simulink model "SOHO_sim_UKF"  (R2018b)
settings: Solver=ode4  StartTime=0.0  StopTime=end_time  FixedStep=dt  RelTol=1e-8  AbsTol=1e-10
undefined symbols (not defined in the file or in its folder): A_RW, acc_gyro, areas, Astar_RW, att_det_method, bcs, DCM, dt, dt_UKF, gyro_noise, I_vec, I_w, mu, mu1, normals, omega, r0, Rot, RW_noise, star_err_var, star_noise, sun_err_var, sun_noise, v0, w0
libraries: sharedutil x1
settings Model: Creator=ayotundedemuren  LastModifiedBy=Ethan
settings SolverCC: AutoScaleAbsTol=off
settings DebuggingCC: UnderSpecifiedDimensionMsg=error

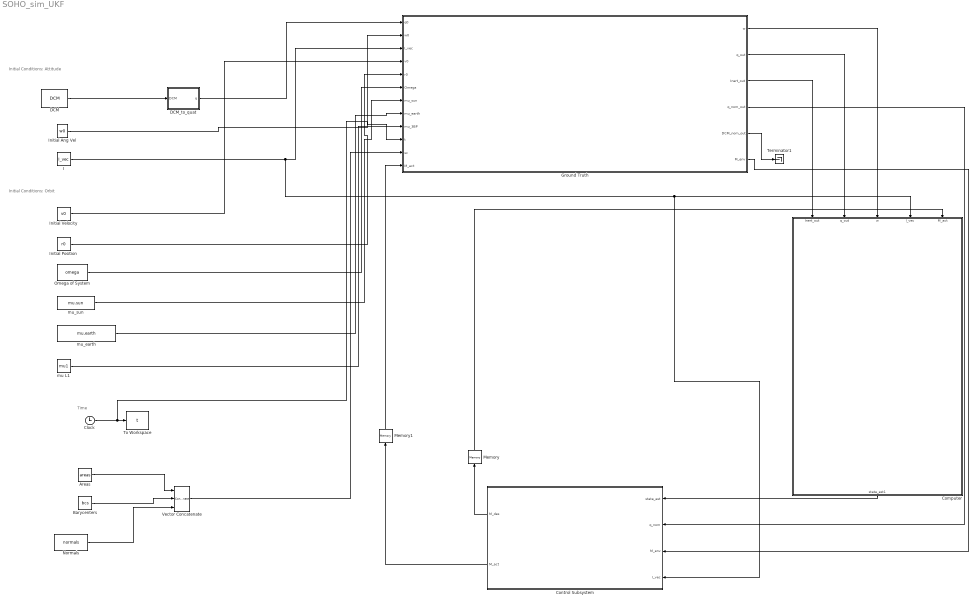
== system SOHO_sim_UKF ==
  note: Time
  note: Initial Conditions: Orbit
  note: Initial Conditions: Attitude
  Areas : Constant  Value=areas
  Barycenters : Constant  Value=bcs
  Clock : Clock
      settings: Decimation=100
  Computer : Subsystem
  Control Subsystem : Subsystem
  DCM : Constant  Value=DCM
  DCM_to_quat : MATLAB Function  TreatAsAtomicUnit=on
  Ground Truth : Subsystem
  I : Constant  Value=I_vec
  Initial Ang Vel : Constant  Value=w0
  Initial Position : Constant  Value=r0
  Initial Velocity : Constant  Value=v0
  Memory : Memory  InitialCondition=zeros(3,1)
  Memory1 : Memory  InitialCondition=zeros(3,1)
  Normals : Constant  Value=normals
  Omega of System : Constant  Value=omega
  Terminator1 : Terminator
  To Workspace : ToWorkspace  VariableName=t  SampleTime=-1
      settings: Save2DSignal=2-D array (concatenate along first dimension)
  Vector Concatenate : Concatenate  NumInputs=3  Mode=Multidimensional array  ConcatenateDimension=2
  mu L1 : Constant  Value=mu1
  mu_earth : Constant  Value=mu.earth
  mu_sun : Constant  Value=mu.sun
  wires:
  Normals/1 -> Vector Concatenate/3
  Barycenters/1 -> Vector Concatenate/2
  Areas/1 -> Vector Concatenate/1
  Clock/1 -> Ground Truth/10(t), To Workspace/1
  DCM/1 -> DCM_to_quat/1(DCM)
  DCM_to_quat/1(q) -> Ground Truth/1(q0)
  Initial Ang Vel/1 -> Ground Truth/2(w0)
  I/1 -> Control Subsystem/4(I_vec), Computer/4(I_vec), Ground Truth/3(I_vec)
  Initial Velocity/1 -> Ground Truth/4(v0)
  Initial Position/1 -> Ground Truth/5(r0)
  Omega of System/1 -> Ground Truth/6(Omega)
  mu_sun/1 -> Ground Truth/7(mu_sun)
  mu_earth/1 -> Ground Truth/8(mu_earth)
  mu L1/1 -> Ground Truth/9(mu_3BP)
  Vector Concatenate/1 -> Ground Truth/11(sc)
  Ground Truth/1(w) -> Computer/3(w)
  Ground Truth/2(q_out) -> Computer/2(q_out)
  Ground Truth/3(Inert_out) -> Computer/1(Inert_out)
  Ground Truth/5(DCM_nom_out) -> Terminator1/1
  Ground Truth/4(q_nom_out) -> Control Subsystem/2(q_nom)
  Control Subsystem/1(M_des) -> Memory/1
  Ground Truth/6(M_env) -> Control Subsystem/3(M_env)
  Memory/1 -> Computer/5(M_act)
  Control Subsystem/2(M_act) -> Memory1/1
  Memory1/1 -> Ground Truth/12(M_act)
  Computer/1(state_est1) -> Control Subsystem/1(state_est)

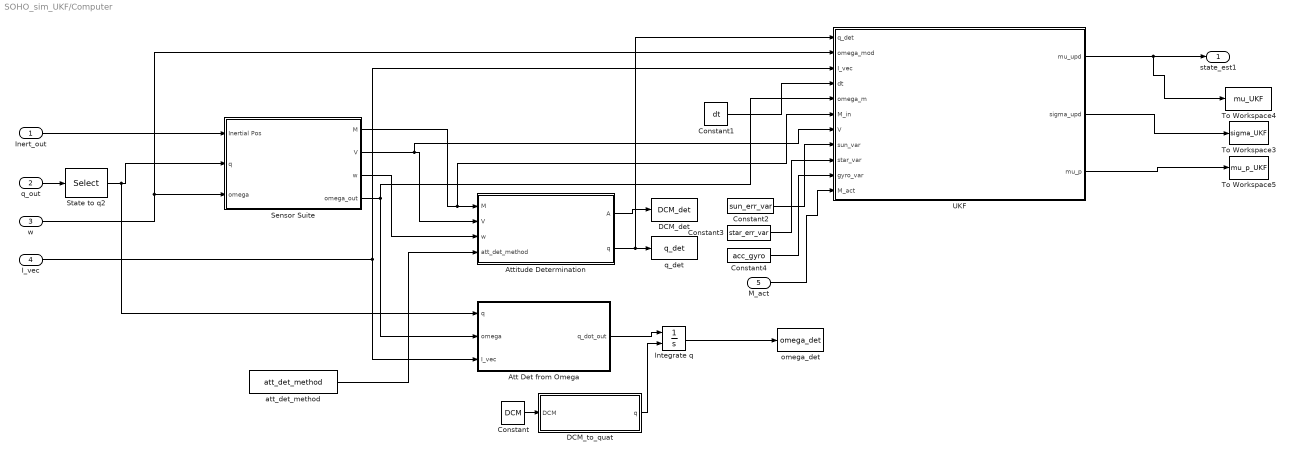
== system SOHO_sim_UKF/Computer ==
  Inert_out : Inport
  q_out : Inport  Port=2
  w : Inport  Port=3
  I_vec : Inport  Port=4
  M_act : Inport  Port=5
  Att Det from Omega : MATLAB Function  TreatAsAtomicUnit=on
  Attitude Determination : MATLAB Function  TreatAsAtomicUnit=on
  Constant : Constant  Value=DCM
  Constant1 : Constant  Value=dt
  Constant2 : Constant  Value=sun_err_var
  Constant3 : Constant  Value=star_err_var
  Constant4 : Constant  Value=acc_gyro
  DCM_det : ToWorkspace  VariableName=DCM_det  SampleTime=-1
  DCM_to_quat : MATLAB Function  TreatAsAtomicUnit=on
  Integrate q : Integrator  InitialConditionSource=external  InitialCondition=DCM(:)
  Sensor Suite : Subsystem
  State to q2 : Selector  InputPortWidth=7  IndexOptions=Starting index (dialog)  Indices=[1]  OutputSizes=4
  To Workspace3 : ToWorkspace  VariableName=sigma_UKF  SampleTime=-1
  To Workspace4 : ToWorkspace  VariableName=mu_UKF  SampleTime=-1
  To Workspace5 : ToWorkspace  VariableName=mu_p_UKF  SampleTime=-1
  UKF : MATLAB Function  TreatAsAtomicUnit=on  SystemSampleTime=dt_UKF
  att_det_method : Constant  Value=att_det_method
  omega_det : ToWorkspace  VariableName=omega_det  SampleTime=-1
  q_det : ToWorkspace  VariableName=q_det  SampleTime=-1
  state_est1 : Outport
  wires:
  Inert_out/1 -> Sensor Suite/1(Inertial Pos)
  q_out/1 -> State to q2/1
  Sensor Suite/1(M) -> UKF/6(M_in), Attitude Determination/1(M)
  Sensor Suite/2(V) -> UKF/7(V), Attitude Determination/2(V)
  att_det_method/1 -> Attitude Determination/4(att_det_method)
  Sensor Suite/3(w) -> Attitude Determination/3(w)
  w/1 -> UKF/2(omega_mod), Sensor Suite/3(omega)
  I_vec/1 -> UKF/3(I_vec), Att Det from Omega/3(I_vec)
  Sensor Suite/4(omega_out) -> UKF/5(omega_m), Att Det from Omega/2(omega)
  Att Det from Omega/1(q_dot_out) -> Integrate q/1
  Attitude Determination/1(A) -> DCM_det/1
  Attitude Determination/2(q) -> UKF/1(q_det), q_det/1
  Constant/1 -> DCM_to_quat/1(DCM)
  DCM_to_quat/1(q) -> Integrate q/2
  Integrate q/1 -> omega_det/1
  State to q2/1 -> Att Det from Omega/1(q), Sensor Suite/2(q)
  Constant1/1 -> UKF/4(dt)
  Constant4/1 -> UKF/10(gyro_var)
  Constant3/1 -> UKF/9(star_var)
  Constant2/1 -> UKF/8(sun_var)
  M_act/1 -> UKF/11(M_act)
  UKF/2(sigma_upd) -> To Workspace3/1
  UKF/3(mu_p) -> To Workspace5/1
  UKF/1(mu_upd) -> To Workspace4/1, state_est1/1

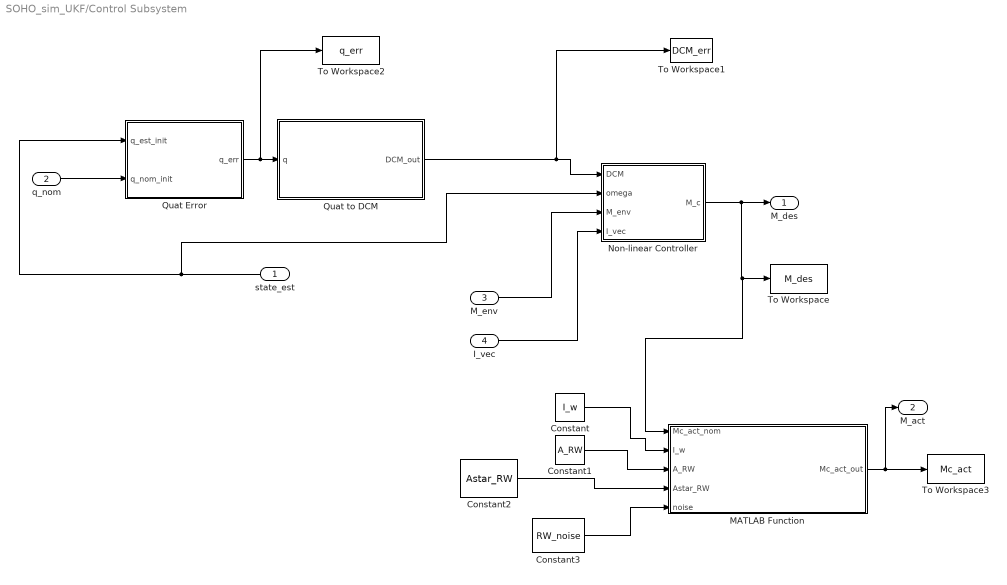
== system SOHO_sim_UKF/Control Subsystem ==
  state_est : Inport
  q_nom : Inport  Port=2
  M_env : Inport  Port=3
  I_vec : Inport  Port=4
  Constant : Constant  Value=I_w
  Constant1 : Constant  Value=A_RW
  Constant2 : Constant  Value=Astar_RW
  Constant3 : Constant  Value=RW_noise
  MATLAB Function : MATLAB Function  TreatAsAtomicUnit=on
  Non-linear Controller : MATLAB Function  TreatAsAtomicUnit=on
  Quat Error : MATLAB Function  TreatAsAtomicUnit=on
  Quat to DCM : MATLAB Function  TreatAsAtomicUnit=on
  To Workspace : ToWorkspace  VariableName=M_des  SampleTime=-1
  To Workspace1 : ToWorkspace  VariableName=DCM_err  SampleTime=-1
  To Workspace2 : ToWorkspace  VariableName=q_err  SampleTime=-1
  To Workspace3 : ToWorkspace  VariableName=Mc_act  SampleTime=-1
  M_des : Outport
  M_act : Outport  Port=2
  wires:
  q_nom/1 -> Quat Error/2(q_nom_init)
  state_est/1 -> Non-linear Controller/2(omega), Quat Error/1(q_est_init)
  Quat Error/1(q_err) -> To Workspace2/1, Quat to DCM/1(q)
  Non-linear Controller/1(M_c) -> MATLAB Function/1(Mc_act_nom), To Workspace/1, M_des/1
  Quat to DCM/1(DCM_out) -> To Workspace1/1, Non-linear Controller/1(DCM)
  M_env/1 -> Non-linear Controller/3(M_env)
  I_vec/1 -> Non-linear Controller/4(I_vec)
  MATLAB Function/1(Mc_act_out) -> M_act/1, To Workspace3/1
  Constant/1 -> MATLAB Function/2(I_w)
  Constant1/1 -> MATLAB Function/3(A_RW)
  Constant2/1 -> MATLAB Function/4(Astar_RW)
  Constant3/1 -> MATLAB Function/5(noise)

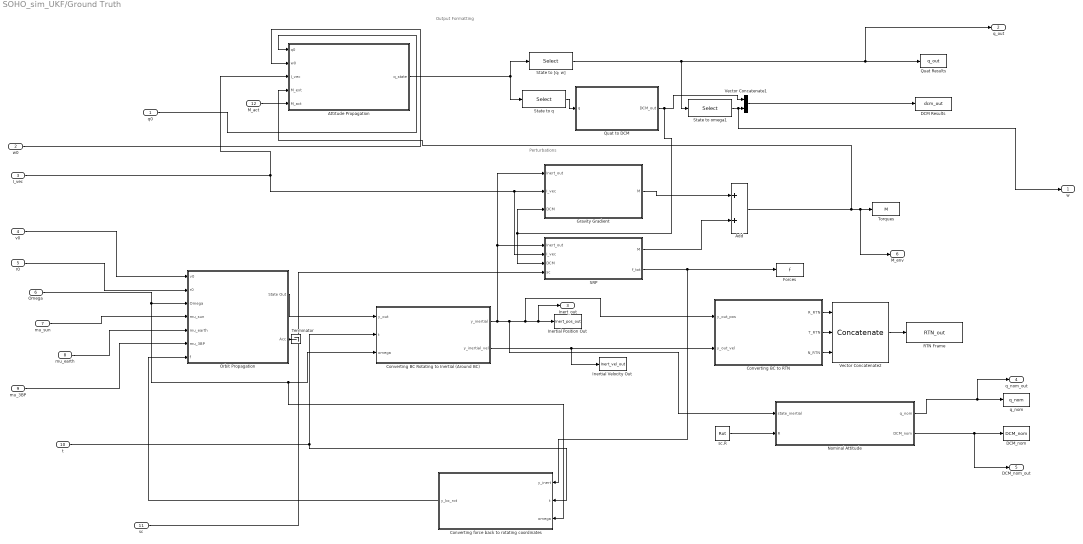
== system SOHO_sim_UKF/Ground Truth ==
  note: Perturbations
  note: Output Formatting
  q0 : Inport
  w0 : Inport  Port=2
  I_vec : Inport  Port=3
  v0 : Inport  Port=4
  r0 : Inport  Port=5
  Omega : Inport  Port=6
  mu_sun : Inport  Port=7
  mu_earth : Inport  Port=8
  mu_3BP : Inport  Port=9
  t : Inport  Port=10
  sc : Inport  Port=11
  M_act : Inport  Port=12
  Add : Sum
  Attitude Propagation : Subsystem
  Converting BC Rotating to Inertial (Around BC) : MATLAB Function  TreatAsAtomicUnit=on
  Converting BC to RTN : MATLAB Function  TreatAsAtomicUnit=on
  Converting force back to rotating coordinates : MATLAB Function  TreatAsAtomicUnit=on
  DCM Results : ToWorkspace  VariableName=dcm_out  SampleTime=-1
      settings: Save2DSignal=2-D array (concatenate along first dimension)
  DCM_nom : ToWorkspace  VariableName=DCM_nom  SampleTime=-1
  Forces : ToWorkspace  VariableName=f  SampleTime=-1
  Gravity Gradient : MATLAB Function  TreatAsAtomicUnit=on
  Inertial Position Out : ToWorkspace  VariableName=Inert_pos_out  SampleTime=-1
  Inertial Velocity Out : ToWorkspace  VariableName=Inert_vel_out  SampleTime=-1
  Nominal Attitude : MATLAB Function  TreatAsAtomicUnit=on
  Orbit Propagation : Subsystem
  Quat Results : ToWorkspace  VariableName=q_out  SampleTime=-1
  Quat to DCM : MATLAB Function  TreatAsAtomicUnit=on
  RTN Frame : ToWorkspace  VariableName=RTN_out  SampleTime=-1
  SRP : MATLAB Function  TreatAsAtomicUnit=on
  State to [q; w] : Selector  InputPortWidth=10  IndexOptions=Starting index (dialog)  Indices=[1]  OutputSizes=7
  State to omega1 : Selector  InputPortWidth=7  IndexOptions=Starting index (dialog)  Indices=5  OutputSizes=3
  State to q : Selector  InputPortWidth=10  IndexOptions=Starting index (dialog)  Indices=[1]  OutputSizes=4
  Terminator : Terminator
  Torques : ToWorkspace  VariableName=M  SampleTime=-1
  Vector Concatenate1 : Concatenate
  Vector Concatenate2 : Concatenate  NumInputs=3  Mode=Multidimensional array  ConcatenateDimension=2
  q_nom : ToWorkspace  VariableName=q_nom  SampleTime=-1
  sc.R : Constant  Value=Rot
  w : Outport
  q_out : Outport  Port=2
  Inert_out : Outport  Port=3
  q_nom_out : Outport  Port=4
  DCM_nom_out : Outport  Port=5
  M_env : Outport  Port=6
  wires:
  Vector Concatenate2/1 -> RTN Frame/1
  State to [q; w]/1 -> State to omega1/1, q_out/1, Quat Results/1
  mu_sun/1 -> Orbit Propagation/4(mu_sun)
  Omega/1 -> Orbit Propagation/3(Omega), Converting force back to rotating coordinates/3(omega), Converting BC Rotating to Inertial (Around BC)/3(omega)
  Vector Concatenate1/1 -> DCM Results/1
  sc/1 -> SRP/4(sc)
  State to q/1 -> Quat to DCM/1(q)
  Quat to DCM/1(DCM_out) -> SRP/3(DCM), Gravity Gradient/3(DCM), Vector Concatenate1/1
  State to omega1/1 -> w/1, Vector Concatenate1/2
  r0/1 -> Orbit Propagation/2(r0)
  Nominal Attitude/1(q_nom) -> q_nom_out/1, q_nom/1
  I_vec/1 -> Attitude Propagation/3(I_vec), SRP/2(I_vec), Gravity Gradient/2(I_vec)
  Converting BC to RTN/1(R_RTN) -> Vector Concatenate2/1
  SRP/2(f_tot) -> Converting force back to rotating coordinates/1(y_inert), Forces/1
  Orbit Propagation/1(State Out) -> Converting BC Rotating to Inertial (Around BC)/1(y_out)
  t/1 -> Converting BC Rotating to Inertial (Around BC)/2(t), Converting force back to rotating coordinates/2(t)
  Converting BC Rotating to Inertial (Around BC)/1(y_inertial) -> SRP/1(Inert_out), Gravity Gradient/1(Inert_out), Nominal Attitude/1(state_inertial), Converting BC to RTN/1(y_out_pos), Inert_out/1, Inertial Position Out/1
  Converting BC Rotating to Inertial (Around BC)/2(y_inertial_vel) -> Inertial Velocity Out/1, Converting BC to RTN/2(y_out_vel)
  q0/1 -> Attitude Propagation/1(q0)
  Converting BC to RTN/2(T_RTN) -> Vector Concatenate2/2
  Converting force back to rotating coordinates/1(y_bc_rot) -> Orbit Propagation/7(f)
  sc.R/1 -> Nominal Attitude/2(R)
  Nominal Attitude/2(DCM_nom) -> DCM_nom_out/1, DCM_nom/1
  v0/1 -> Orbit Propagation/1(v0)
  SRP/1(M) -> Add/2
  Attitude Propagation/1(q_state) -> State to [q; w]/1, State to q/1
  Gravity Gradient/1(M) -> Add/1
  Converting BC to RTN/3(N_RTN) -> Vector Concatenate2/3
  w0/1 -> Attitude Propagation/2(w0)
  mu_3BP/1 -> Orbit Propagation/6(mu_3BP)
  mu_earth/1 -> Orbit Propagation/5(mu_earth)
  Orbit Propagation/2(Acc) -> Terminator/1
  Add/1 -> Attitude Propagation/4(M_ext), M_env/1, Torques/1
  M_act/1 -> Attitude Propagation/5(M_act)

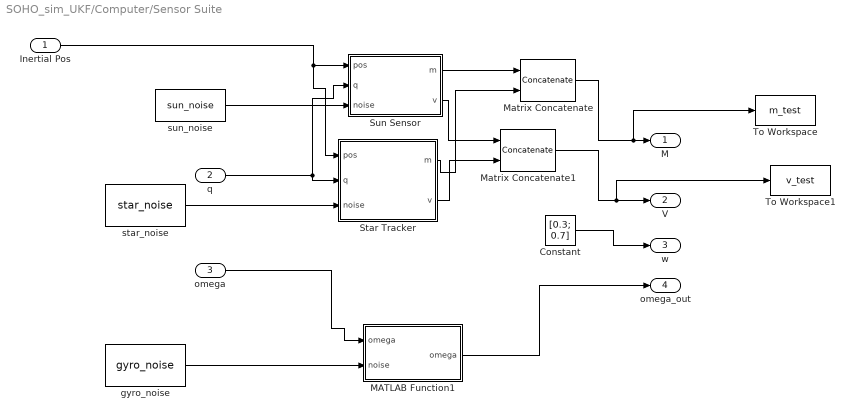
== system SOHO_sim_UKF/Computer/Sensor Suite ==
  Inertial Pos : Inport
  q : Inport  Port=2
  omega : Inport  Port=3
  Constant : Constant  Value=[0.3; 0.7]  VectorParams1D=off
  MATLAB Function1 : MATLAB Function  TreatAsAtomicUnit=on  SystemSampleTime=dt
  Matrix Concatenate : Concatenate  Mode=Multidimensional array  ConcatenateDimension=2
  Matrix Concatenate1 : Concatenate  Mode=Multidimensional array  ConcatenateDimension=2
  Star Tracker : MATLAB Function  TreatAsAtomicUnit=on  SystemSampleTime=dt
  Sun Sensor : MATLAB Function  TreatAsAtomicUnit=on  SystemSampleTime=dt
  To Workspace : ToWorkspace  VariableName=m_test  SampleTime=-1
  To Workspace1 : ToWorkspace  VariableName=v_test  SampleTime=-1
  gyro_noise : Constant  Value=gyro_noise  VectorParams1D=off
  star_noise : Constant  Value=star_noise  VectorParams1D=off
  sun_noise : Constant  Value=sun_noise  VectorParams1D=off
  M : Outport
  V : Outport  Port=2
  w : Outport  Port=3
  omega_out : Outport  Port=4
  wires:
  Inertial Pos/1 -> Star Tracker/1(pos), Sun Sensor/1(pos)
  q/1 -> Sun Sensor/2(q), Star Tracker/2(q)
  omega/1 -> MATLAB Function1/1("omega ")
  Sun Sensor/1(m) -> Matrix Concatenate/1
  Star Tracker/1(m) -> Matrix Concatenate/2
  Matrix Concatenate/1 -> To Workspace/1, M/1
  Sun Sensor/2(v) -> Matrix Concatenate1/1
  Star Tracker/2(v) -> Matrix Concatenate1/2
  Matrix Concatenate1/1 -> To Workspace1/1, V/1
  Constant/1 -> w/1
  MATLAB Function1/1(omega) -> omega_out/1
  sun_noise/1 -> Sun Sensor/3(noise)
  star_noise/1 -> Star Tracker/3(noise)
  gyro_noise/1 -> MATLAB Function1/2(noise)

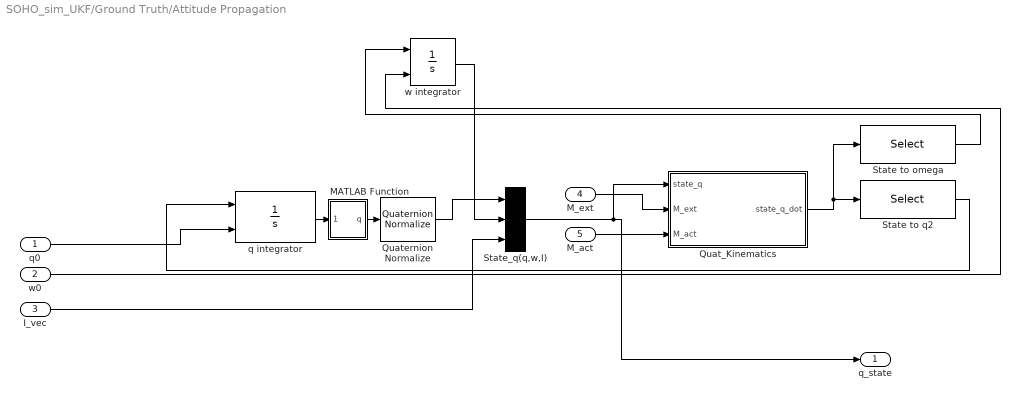
== system SOHO_sim_UKF/Ground Truth/Attitude Propagation ==
  q0 : Inport
  w0 : Inport  Port=2
  I_vec : Inport  Port=3
  M_ext : Inport  Port=4
  M_act : Inport  Port=5
  MATLAB Function : MATLAB Function  TreatAsAtomicUnit=on
  Quat_Kinematics : MATLAB Function  TreatAsAtomicUnit=on
  Quaternion Normalize : sharedutil/Quaternion Normalize  aMode=aMode
      settings: SourceProductName=Aerospace Blockset  SourceProductBaseCode=AE
  State to omega : Selector  InputPortWidth=10  IndexOptions=Starting index (dialog)  Indices=5  OutputSizes=3
  State to q2 : Selector  InputPortWidth=10  IndexOptions=Starting index (dialog)  Indices=[1]  OutputSizes=4
  State_q(q,w,I) : Concatenate  NumInputs=3
  q integrator : Integrator  InitialConditionSource=external
  w integrator : Integrator  InitialConditionSource=external
  q_state : Outport
  wires:
  State_q(q,w,I)/1 -> q_state/1, Quat_Kinematics/1(state_q)
  w integrator/1 -> State_q(q,w,I)/2
  State to omega/1 -> w integrator/1
  Quat_Kinematics/1(state_q_dot) -> State to omega/1, State to q2/1
  State to q2/1 -> q integrator/1
  w0/1 -> w integrator/2
  q0/1 -> q integrator/2
  I_vec/1 -> State_q(q,w,I)/3
  M_ext/1 -> Quat_Kinematics/2(M_ext)
  M_act/1 -> Quat_Kinematics/3(M_act)
  Quaternion Normalize/1 -> State_q(q,w,I)/1
  q integrator/1 -> MATLAB Function/1(q_in)
  MATLAB Function/1(q) -> Quaternion Normalize/1

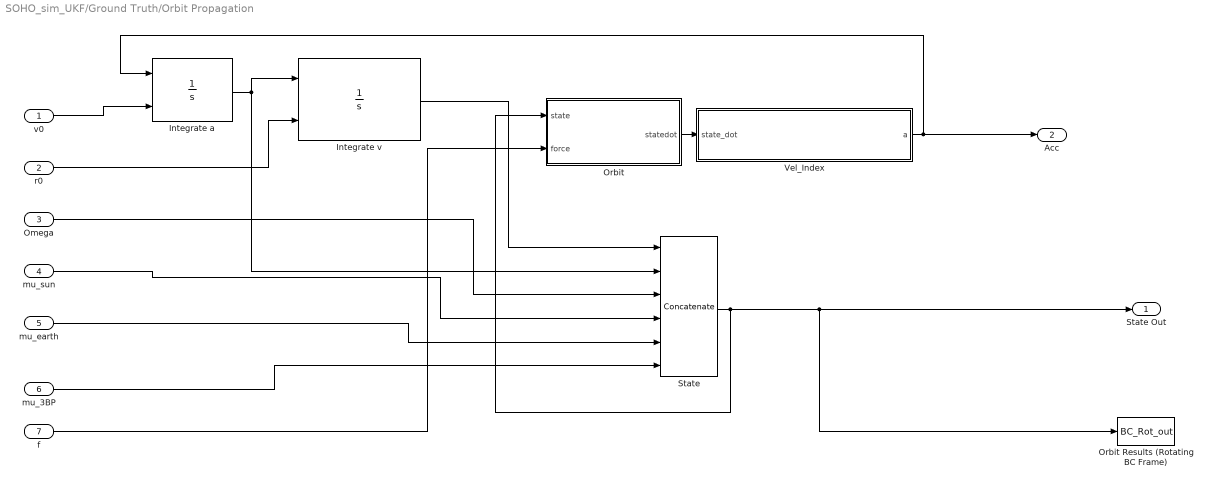
== system SOHO_sim_UKF/Ground Truth/Orbit Propagation ==
  v0 : Inport
  r0 : Inport  Port=2
  Omega : Inport  Port=3
  mu_sun : Inport  Port=4
  mu_earth : Inport  Port=5
  mu_3BP : Inport  Port=6
  f : Inport  Port=7
  Integrate a : Integrator  InitialConditionSource=external  AbsoluteTolerance=1e-6
  Integrate v : Integrator  InitialConditionSource=external  AbsoluteTolerance=1e-6
  Orbit : MATLAB Function  TreatAsAtomicUnit=on
  Orbit Results (Rotating BC Frame) : ToWorkspace  VariableName=BC_Rot_out  SampleTime=-1
  "State " : Concatenate  NumInputs=6
  Vel_Index : MATLAB Function  TreatAsAtomicUnit=on
  State Out : Outport
  Acc : Outport  Port=2
  wires:
  r0/1 -> Integrate v/2
  Integrate a/1 -> "State "/2, Integrate v/1
  Integrate v/1 -> "State "/1
  "State "/1 -> Orbit/1(state), Orbit Results (Rotating BC Frame)/1, State Out/1
  Vel_Index/1(a) -> Integrate a/1, Acc/1
  Orbit/1(statedot) -> Vel_Index/1(state_dot)
  v0/1 -> Integrate a/2
  mu_3BP/1 -> "State "/6
  Omega/1 -> "State "/3
  mu_sun/1 -> "State "/4
  mu_earth/1 -> "State "/5
  f/1 -> Orbit/2(force)

== matlab function SOHO_sim_UKF/Ground Truth/Orbit Propagation/Vel_Index ==
  data: state_dot input; a output
function a = fcn(state_dot)

a = state_dot(4:6);

end

== matlab function SOHO_sim_UKF/Ground Truth/Orbit Propagation/Orbit ==
  data: state input; statedot output; force input
function statedot = fcn(state, force)
force = force*0;
dis_sun = 149599650;

statedot = zeros(length(state),1);
x = state(1);
y = state(2);
z = state(3);
xdot = state(4);
ydot = state(5);
zdot = state(6);

w = state(7);
mu1 = state(8);
mu2 = state(9);
mu_sys = state(10);

Rx1 = - mu_sys*dis_sun;
Rx2 = (1-mu_sys)*dis_sun;

R1 = sqrt((x - Rx1)^2 + y^2 + z^2);
R2 = sqrt((x - Rx2)^2 + y^2 + z^2);

statedot(1) = xdot;
statedot(2) = ydot;
statedot(3) = zdot;

statedot(4) = x*w^2 + 2*ydot*w + mu1 * (Rx1 - x)/R1^3 + mu2 * (Rx2 - x)/R2^3 + force(1);
statedot(5) = y*w^2 - 2*xdot*w - mu1 * (y)/R1^3 - mu2 * (y)/R2^3 + force(2);
statedot(6) = - mu1 * (z)/R1^3 - mu2 * (z)/R2^3 + force(3);
end

== matlab function SOHO_sim_UKF/Ground Truth/Converting BC to RTN ==
  data: y_out_pos input; R_RTN output; T_RTN output; N_RTN output; y_out_vel input
function [R_RTN, T_RTN, N_RTN] = BCRot_to_RTN(y_out_pos, y_out_vel)
% 
% %% RTN Frame Rotating
% r = y_out(1:3);
% v = y_out(4:6);
% R_RTN = zeros(3,1);
% T_RTN = zeros(3,1);
% N_RTN = zeros(3,1);
% 
% for ii = 1:1
% 
%     R_RTN = r ./ norm(r);
%     N_RTN = cross(r,v) ./norm(cross(r,v));
%     T_RTN = cross(N_RTN, R_RTN) ./ norm(cross(N_RTN, R_RTN));
% end

%% RTN Frame Inertial
r = y_out_pos(1:3);
v = y_out_vel(1:3);
R_RTN = zeros(3,1);
T_RTN = zeros(3,1);
N_RTN = zeros(3,1);

for ii = 1:1

    R_RTN = r ./ norm(r);
    N_RTN = cross(r,v) ./norm(cross(r,v));
    T_RTN = cross(N_RTN, R_RTN) ./ norm(cross(N_RTN, R_RTN));
end
end

== matlab function SOHO_sim_UKF/Ground Truth/Converting BC Rotating to Inertial (Around BC) ==
  data: y_out input; y_inertial output; t input; omega input; y_inertial_vel output
function [y_inertial, y_inertial_vel] = BCRot_to_Inertial(y_out, t, omega)
wt = omega * t;
R = zeros(3,3);
R(1,:) = [cos(wt) sin(wt) 0];
R(2,:) = [-sin(wt) cos(wt) 0];
R(3,:) = [0 0 1];

sun_init = [-4.548476597303452e+02; 0; 0];
earth_init = [1.495991951523403e+08; 0; 0];
y_inertial = zeros(9, 1);
y_inertial_vel = zeros(9, 1);

y_inertial(1:3) = R' * y_out(1:3);
y_inertial_vel(1:3) = R' * y_out(4:6) + cross([0; 0; omega], y_inertial(1:3));
y_inertial(4:6) = R' * sun_init;
y_inertial_vel(4:6) = cross([0; 0; omega], y_inertial(4:6));
y_inertial(7:9) = R' * earth_init;
y_inertial_vel(7:9) = cross([0; 0; omega], y_inertial(7:9));
end

== matlab function SOHO_sim_UKF/Ground Truth/Attitude Propagation/Quat_Kinematics ==
  data: state_q input; state_q_dot output; M_ext input; M_act input
function state_q_dot  = quat_kin(state_q, M_ext, M_act)
% state = [q1 q2 q3 q4 w1 w2 w3 I1 I2 I3]

state_q_dot = zeros(length(state_q),1);
wx = state_q(5);
wy = state_q(6);
wz = state_q(7);
%% Kinematic Equations
Omega = [0 wz -wy wx; -wz 0 wx wy; wy -wx 0 wz; -wx -wy -wz 0];
err = 1 - norm(state_q(1:4));
state_q_dot(1:4) = 1/2 * Omega * state_q(1:4) + 0.05 * err * state_q(1:4);

%% Euler Equations
state_q_dot(5:end) = euler_eq(state_q(5:end), M_ext, M_act);
% state_q_dot(5) = -wy*wz * (state_q(10) - state_q(9))/state_q(8);
% state_q_dot(6) = -wx*wz * (state_q(8) - state_q(10))/state_q(9);
% state_q_dot(7) = -wx*wy * (state_q(9) - state_q(8))/state_q(10);

end

== matlab function SOHO_sim_UKF/DCM_to_quat ==
  data: DCM input; q output
function q  = DCM_to_quat(DCM)
B4 = 1/4 * (1 + trace(DCM));
B1 = 1/4 * (1 + 2*DCM(1,1) - trace(DCM));
B2 = 1/4 * (1 + 2*DCM(2,2) - trace(DCM));
B3 = 1/4 * (1 + 2*DCM(3,3) - trace(DCM));
B = [B1 B2 B3 B4];
[M, I] = max(B);
q = zeros(4,1);

q(I) = sqrt(B(I));
if I == 4
    q(1) = (DCM(2,3) - DCM(3,2)) / 4 / q(I);
    q(2) = (DCM(3,1) - DCM(1,3)) / 4 / q(I);
    q(3) = (DCM(1,2) - DCM(2,1)) / 4 / q(I);
elseif I == 3
  
    q(2) = (DCM(2,3) + DCM(3,2)) / 4 / q(I);
    q(1) = (DCM(3,1) + DCM(1,3)) / 4 / q(I);
    q(4) = (DCM(1,2) - DCM(2,1)) / 4 / q(I);
elseif I == 2

    q(3) = (DCM(2,3) + DCM(3,2)) / 4 / q(I);
    q(4) = (DCM(3,1) - DCM(1,3)) / 4 / q(I);
    q(1) = (DCM(1,2) + DCM(2,1)) / 4 / q(I);
elseif I == 1
    q(4) = (DCM(2,3) - DCM(3,2)) / 4 / q(I);
    q(3) = (DCM(3,1) + DCM(1,3)) / 4 / q(I);
    q(2) = (DCM(1,2) + DCM(2,1)) / 4 / q(I);
end
q = q/norm(q);
end

== matlab function SOHO_sim_UKF/Ground Truth/Gravity Gradient ==
  data: Inert_out input; M output; I_vec input; DCM input
function M = grav_grad(Inert_out, I_vec, DCM)
% Inert_out = [sat; sun; earth]

x = Inert_out(1);
y = Inert_out(2);
z = Inert_out(3);

x_s = Inert_out(4);
y_s = Inert_out(5);
z_s = Inert_out(6);

x_e = Inert_out(7);
y_e = Inert_out(8);
z_e = Inert_out(9);

Ix_sat = I_vec(1);
Iy_sat = I_vec(2);
Iz_sat = I_vec(3);

R_s = sqrt(((x - x_s).^2)+((y - y_s).^2)+((z - z_s).^2));
R_e = sqrt(((x - x_e).^2)+((y - y_e).^2)+((z - z_e).^2));

[A] = out2mat(DCM);
c_vec_s = A * [x-x_s; y-y_s; z-z_s];
cx_s = c_vec_s(1)/R_s;
cy_s = c_vec_s(2)/R_s;
cz_s = c_vec_s(3)/R_s;

c_vec_e = A * [x-x_e; y-y_e; z-z_e];
cx_e = c_vec_e(1)/R_e;
cy_e = c_vec_e(2)/R_e;
cz_e = c_vec_e(3)/R_e;

mu_earth = 3.986004418000000e+05;
mu_sun =  1.327124400180000e+11;

M_earth = (3*mu_earth./(R_e.^3)).*[((Iz_sat - Iy_sat).*cy_e.*cz_e)';...
    ((Ix_sat - Iz_sat).*cz_e.*cx_e)';...
    ((Iy_sat - Ix_sat).*cx_e.*cy_e)'];

M_sun = (3*mu_sun./(R_s.^3)).*[((Iz_sat - Iy_sat).*cy_s.*cz_s)';...
    ((Ix_sat - Iz_sat).*cz_s.*cx_s)';...
    ((Iy_sat - Ix_sat).*cx_s.*cy_s)'];

M = M_earth + M_sun;

== matlab function SOHO_sim_UKF/Ground Truth/Quat to DCM ==
  data: q input; DCM_out output
function DCM_out  = quat_to_DCM(q)

DCM = zeros(3, 3);
DCM(:, :) = ((q(4)^2 - norm(q(1:3))^2)*eye(3) ...
    + 2 * q(1:3) * q(1:3)'...
    - 2 * q(4) * ...
    [0, -q(3), q(2); q(3), 0, -q(1); ...
    -q(2), q(1), 0]);

DCM_out = DCM(:)';
end

== matlab function SOHO_sim_UKF/Ground Truth/Converting force back to rotating coordinates ==
  data: y_inert input; y_bc_rot output; t input; omega input
function y_bc_rot  = Inertial_to_BCRot(y_inert, t, omega)
wt = omega * t;
R = zeros(3,3);
R(1,:) = [cos(wt) sin(wt) 0];
R(2,:) = [-sin(wt) cos(wt) 0];
R(3,:) = [0 0 1];

y_bc_rot = zeros(3, 1);

y_bc_rot(1:3) = R * y_inert(1:3);

end

== matlab function SOHO_sim_UKF/Ground Truth/Nominal Attitude ==
  data: state_inertial input; q_nom output; DCM_nom output; R input
function [q_nom, DCM_nom] = nominal(state_inertial, R)
sat_pos = state_inertial(1:3);
sun_pos = state_inertial(4:6);

vect_to_sun = (sun_pos - sat_pos) / norm((sun_pos - sat_pos));
b_x = vect_to_sun;
b_y = cross([0; 0; 1], b_x);
b_z = cross(b_x, b_y);

DCM_nom_temp = R'*[b_x'; b_y'; b_z'];
q_nom = DCM_to_quat(DCM_nom_temp);

DCM_nom = DCM_nom_temp(:);


end

== matlab function SOHO_sim_UKF/Computer/Attitude Determination ==
  data: M input; A output; V input; w input; att_det_method input; q output
function [A, q] = att_det(M, V, w, att_det_method)

A = eye(3);
q = [0;0;0;1];
if att_det_method == 0
    A = det_method(M, V);
    q = DCM_to_quat(A);
    
elseif att_det_method == 1
    W = zeros(3, length(w));
    V2 = zeros(3, length(w));
    for ii = 1:length(w)
        W(:, ii) = sqrt(w(ii)).*M(:, ii);
        V2(:, ii) = sqrt(w(ii)).*V(:, ii);
    end
    [A, q] = q_method(W, V2);
    
elseif att_det_method == 2
    A = eye(3);
    q = ones(4,1);
end

end

== matlab function SOHO_sim_UKF/Computer/Sensor Suite/Sun Sensor ==
  data: pos input; m output; q input; v output; noise input
function [m, v] = sun_sens(pos, q, noise)
% Basic sun sensor
persistent count;
if isempty(count)
    count = 1;
elseif count >= size(noise, 2)
    count = 1;
    noise = [noise(3,:); -noise(1, :); noise(2, :)];
end


q = q(1:4);
A = quat_to_DCM(q);
v = (pos(4:6) - pos(1:3)) / norm((pos(4:6) - pos(1:3))); % sun to sat vec
m = A * v + noise(:, count); % currently this will give the exact measurement back 
count = count + 1;

end

== matlab function SOHO_sim_UKF/Computer/Att Det from Omega ==
  data: q input; omega input; q_dot_out output; I_vec input
function q_dot_out = fcn(q, omega, I_vec)
A = quat_to_DCM(q);
state = [q; omega; I_vec];
t = 1;
[state_dot] = quat_kin(t, state);
q_dot_out = state_dot(1:4);
end

== matlab function SOHO_sim_UKF/Computer/Sensor Suite/Star Tracker ==
  data: pos input; m output; q input; v output; noise input
function [m, v] = star_track(pos, q, noise)

persistent count;
if isempty(count)
    count = 1;
elseif count >= size(noise, 2)
    count = 1;
    noise = [noise(3,:); noise(1, :); noise(2, :)];
end

A = quat_to_DCM(q);
v = [0; 0; 1]; % star is in direction straight above satellite in inertial
% not too bad of an assumption since it is so far away that it will remain
% nearly constant overhead for now
m = A * v + noise(:, count); % currently this will give the exact measurement back 

count = count + 1;

end

== matlab function SOHO_sim_UKF/Computer/DCM_to_quat ==
  data: DCM input; q output
function q  = DCM_to_quat(DCM)
B4 = 1/4 * (1 + trace(DCM));
B1 = 1/4 * (1 + 2*DCM(1,1) - trace(DCM));
B2 = 1/4 * (1 + 2*DCM(2,2) - trace(DCM));
B3 = 1/4 * (1 + 2*DCM(3,3) - trace(DCM));
B = [B1 B2 B3 B4];
[M, I] = max(B);
q = zeros(4,1);
% q(4) = sqrt(B(I));
q(I) = sqrt(B(I));
if I == 4
    q(1) = (DCM(2,3) - DCM(3,2)) / 4 / q(I);
    q(2) = (DCM(3,1) - DCM(1,3)) / 4 / q(I);
    q(3) = (DCM(1,2) - DCM(2,1)) / 4 / q(I);
elseif I == 3
%     q(2) = (DCM(2,3) + DCM(3,2)) / 4 / q(4);
%     q(1) = (DCM(3,1) + DCM(1,3)) / 4 / q(4);
%     q(3) = (DCM(1,2) - DCM(2,1)) / 4 / q(4);
    
    q(2) = (DCM(2,3) + DCM(3,2)) / 4 / q(I);
    q(1) = (DCM(3,1) + DCM(1,3)) / 4 / q(I);
    q(4) = (DCM(1,2) - DCM(2,1)) / 4 / q(I);
elseif I == 2
%     q(2) = (DCM(2,3) + DCM(3,2)) / 4 / q(4);
%     q(3) = (DCM(3,1) - DCM(1,3)) / 4 / q(4);
%     q(1) = (DCM(1,2) + DCM(2,1)) / 4 / q(4);
    q(3) = (DCM(2,3) + DCM(3,2)) / 4 / q(I);
    q(4) = (DCM(3,1) - DCM(1,3)) / 4 / q(I);
    q(1) = (DCM(1,2) + DCM(2,1)) / 4 / q(I);
elseif I == 1
%     q(3) = (DCM(2,3) - DCM(3,2)) / 4 / q(4);
%     q(2) = (DCM(3,1) + DCM(1,3)) / 4 / q(4);
%     q(1) = (DCM(1,2) + DCM(2,1)) / 4 / q(4);
    q(4) = (DCM(2,3) - DCM(3,2)) / 4 / q(I);
    q(3) = (DCM(3,1) + DCM(1,3)) / 4 / q(I);
    q(2) = (DCM(1,2) + DCM(2,1)) / 4 / q(I);
end
q = q/norm(q);
end

== matlab function SOHO_sim_UKF/Ground Truth/SRP ==
  data: Inert_out input; M output; I_vec input; DCM input; sc input; f_tot output
function [M,f_tot] = SRP(Inert_out, I_vec, DCM,sc)

F = 1358; % solar constant
c = 3e8;
P = F/c;
% sc data
areas = sc(1:end,1);
bcs = sc(1:end,2:4);
normals = sc(1:end,5:7);
% Principal Moments of Inertia
Ix_sat = I_vec(1);
Iy_sat = I_vec(2);
Iz_sat = I_vec(3);
% Inertial Sat Coordinates
x = Inert_out(1);
y = Inert_out(2);
z = Inert_out(3);
% Inertial Sun Coordinates
x_s = Inert_out(4);
y_s = Inert_out(5);
z_s = Inert_out(6);
% DCM
[A] = out2mat(DCM);
% Relative Sun to Sat Vector

r_sat2s = [x_s-x,y_s-y,z_s-z]; % vector
R_s2s = sqrt((r_sat2s(1).^2)+(r_sat2s(2).^2)+(r_sat2s(3).^2)); % magnitude
r_sp = A*r_sat2s'; % sun vector in principal frame
r_sp_hat = r_sp./R_s2s;

% SRP Coefficients
C_a = 0.1;
C_s = 0.2;
C_d = 0.7;

% initialize
M = [0,0,0]';
f = [0,0,0]';
f_tot = zeros(3,1);
r_press = zeros(3,1);
s_hat = r_sp_hat;

% Calculate SRP Force and Moment
for i = 1:length(areas)
    bc = bcs(i,:);
    area = areas(i);
    normal = normals(i,:);
    r_press = bc';
    n_hat = normal';
%     theta = atan2d(norm(cross(s_hat,n_hat)),dot(s_hat,n_hat));
    theta = acosd(dot(s_hat,n_hat));
    if dot(n_hat,s_hat) > 0 
        f = -P * area * cosd(theta)*((1-C_s)*s_hat + 2*(C_s*cosd(theta)+1/3*C_d)*n_hat);
        f_tot = f_tot + f;
        M = M + cross(r_press,f);
    else
    end
end

== matlab function SOHO_sim_UKF/Computer/Sensor Suite/MATLAB Function1 ==
  data: omega input; omega output; noise input
function omega = gyro(omega, noise)


persistent count;
if isempty(count)
    count = 1;
elseif count >= size(noise, 2)
    count = 1;
    noise = [noise(3,:); noise(1, :); noise(2, :)];
end

% acc_gyro = 1e6 * pi/180 / 60 / 60; %0.001 deg/hr (SMAD)
% noise = randn(1,3)*chol(eye(3)*acc_gyro);
% omega = omega;
omega = omega + noise(:, count);

count = count + 1;
end

== matlab function SOHO_sim_UKF/Control Subsystem/Quat Error ==
  data: q_est_init input; q_err output; q_nom_init input
function q_err = quat_error(q_est_init, q_nom_init)
[q_est] = quat_corr(q_est_init(1:4)');
[q_nom] = quat_corr(q_nom_init(1:4)');
q_mat = [q_nom(4) q_nom(3) -q_nom(2) q_nom(1);...
        -q_nom(3) q_nom(4) q_nom(1) q_nom(2);...
        q_nom(2) -q_nom(1) q_nom(4) q_nom(3);...
        -q_nom(1) -q_nom(2) -q_nom(3) q_nom(4)];

q_err = q_mat * [-q_est(1) -q_est(2) -q_est(3) q_est(4)]';
q_err = quat_corr(q_err')';
end

== matlab function SOHO_sim_UKF/Control Subsystem/Quat to DCM ==
  data: q input; DCM_out output
function DCM_out  = quat_to_DCM(q)

DCM_out = zeros(3, 3);
DCM_out(:, :) = ((q(4)^2 - norm(q(1:3))^2)*eye(3) ...
    + 2 * q(1:3) * q(1:3)'...
    - 2 * q(4) * ...
    [0, -q(3), q(2); q(3), 0, -q(1); ...
    -q(2), q(1), 0]);

end

== matlab function SOHO_sim_UKF/Ground Truth/Attitude Propagation/MATLAB Function ==
  data: q_in input; q output
function q  = quat_corr(q_in)
q = q_in';
for ii = 1:size(q, 1)
    if q(ii, 4) < 0
        q(ii, 1:4) = q(ii, 1:4) * -1;
    end
end
% q = q';
end

== matlab function SOHO_sim_UKF/Control Subsystem/Non-linear Controller ==
  data: DCM input; M_c output; omega input; M_env input; I_vec input
function M_c = controller(DCM, omega, M_env, I_vec)
w = omega(5:7);
M_c = zeros(3, 1);
M_env = ones(3, 1) * 7.363003685852291e-05;
kp = 60^2 ./ (I_vec);
kd = zeros(3,1);
% kd = 2 * sqrt(diag(I_vec) .* (M_env + kp));
kd(1) = 2 * sqrt(I_vec(1) .* abs(M_env(1) + kp(1)));
kd(2) = 2 * sqrt(I_vec(2) .* abs(M_env(2) + kp(2)));
kd(3) = 2 * sqrt(I_vec(3) .* abs(M_env(3) + kp(3)));

M_c(1) = -kp(1) * (DCM(2, 3) - DCM(3, 2))/2 - kd(1) * w(1);
M_c(2) = -kp(2) * (DCM(3, 1) - DCM(1, 3))/2 - kd(2) * w(2);
M_c(3) = -kp(3) * (DCM(1, 2) - DCM(2, 1))/2 - kd(3) * w(3);
M_c = M_c * -1;
% M_c = M_c * 0;
% M_c = min(max(M_c, -0.2), 0.2);
M_c = min(max(M_c, -1), 1);
end

== matlab function SOHO_sim_UKF/Control Subsystem/MATLAB Function ==
  settings: updateMethod=DISCRETE
  data: Mc_act_nom input; Mc_act_out output; I_w input; A_RW input; Astar_RW input; noise input
function Mc_act_out  = RW_M(Mc_act_nom,I_w,A_RW,Astar_RW,noise)
% Initialization
L_w_dot = zeros(4,1);
w_dot = zeros(4,1);
Mc_act_out = zeros(3,1);
% Generate noise
persistent count;
if isempty(count)
    count = 1;
elseif count >= size(noise, 2)
    count = 1;
    noise = [noise(3,:); -noise(1, :); -noise(4, :); noise(2, :)];
end

% Reaction wheel model
L_w_dot = Astar_RW*Mc_act_nom;
w_dot = I_w \ L_w_dot;
w_dot = w_dot + noise(:, count);
Mc_act_out = A_RW*I_w*w_dot;
Mc_act_out = min(max(Mc_act_out, -1), 1);
count = count + 1;

== matlab function SOHO_sim_UKF/Computer/UKF ==
  data: q_det input; omega_mod input; mu_upd output; I_vec input; dt input; sigma_upd output; omega_m input; M_in input; V input; sun_var input; star_var input; gyro_var input; mu_p output; M_act input
function [mu_upd, sigma_upd, mu_p] = UKF(q_det, omega_mod, I_vec, dt, ...
    omega_m, M_in, V, sun_var, star_var, gyro_var, M_act)
%% Dynamics Initialization
persistent sigma_prev
persistent mu_prev
if isempty(mu_prev)
    mu_prev = zeros(7, 1);
    mu_prev(1:4) = [q_det(1); q_det(2); q_det(3); q_det(4)];
    mu_prev(5:7) = [omega_mod(1); omega_mod(2); omega_mod(3)];
end
q = mu_prev(1:4);
w = mu_prev(5:7);

% Qt = eye(7).*1e-5;
Qt = diag([1e-5*ones(1,4), 1e-2 * ones(1,3)]);
sigma0 = eye(7) * 1;
lambda = 4;

gyro_flag = 1; % leave this as 1 for now, can switch to 0 if gyros break!
%% Measurement Initialization
% Measurement Model
M = M_in;
if gyro_flag == 1
    M = [M_in omega_m];
else
    M = M_in;
end
yt = zeros(size(M, 2) * 3, 1);
% Measurement model
for ii = 1:size(M, 2)
    yt(1 + 3 * (ii -1): 3 + 3 * (ii -1), 1) = M(:, ii);
end
%% Estimated measurements
Rt = diag([sun_var*ones(1,3) star_var*ones(1,3) gyro_var*ones(1,3)]);
Rt = Rt(1:size(M, 2)*3, 1:size(M, 2)*3);
%% UKF, Predict
if isempty(sigma_prev)
   sigma_prev = sigma0;
end


[x_p, w_p] = UT(mu_prev, sigma_prev, lambda);
x_p_bar = zeros(size(x_p));
t = 1; %dummy variable
for ii = 1:size(x_p, 2)
    state = [x_p(:, ii); I_vec];
    [state_dot] = quat_kin_EKF(t, state, M_act);
    x_p_bar(:, ii) = x_p(:, ii) + dt * state_dot(1:7);
    x_p_bar(1:4, ii) = x_p_bar(1:4, ii) ./ norm(x_p_bar(1:4, ii));
end

[mu_p, sigma_bar] = UT_inv(x_p_bar, w_p);
mu_p(1:4) = mu_p(1:4) ./ norm(mu_p(1:4));
sigma_p = sigma_bar + Qt;

%% UKF, Update
[x_p, w_p] = UT(mu_p, sigma_p, lambda);
y_fake = zeros(size(x_p, 2), 3 * size(M, 2));
y_hat = zeros(3 * size(M, 2), 1);
for ii = 1:size(x_p, 2)
    A = quat_to_DCM(x_p(1:4, ii));
    for jj = 1:size(V, 2)
        y_fake(ii, 1 + 3 * (jj - 1): 3 + 3 * (jj - 1)) = measurement_model_vector(A, V(:, jj))';
        y_hat(1 + 3 * (jj - 1): 3 + 3 * (jj - 1), 1) = ...
            y_hat(1 + 3 * (jj - 1): 3 + 3 * (jj - 1), 1) + w_p(ii) ...
                * y_fake(ii, 1 + 3 * (jj - 1): 3 + 3 * (jj - 1))';
    end
    if gyro_flag == 1
        y_fake(ii, 1 + 3 * size(V,2): 3 + 3 * size(V,2)) = x_p(5:7, ii)';
        y_hat(1 + 3 * size(V,2): 3 + 3 * size(V,2), 1) = ... 
                y_hat(1 + 3 * size(V,2): 3 + 3 * size(V,2), 1) + ...
                    w_p(ii) * ...
                    y_fake(ii, 1 + 3 * size(V,2): 3 + 3 * size(V,2))';
    end
end

E_y = zeros(size(y_hat, 1), size(y_hat, 1));
E_xy = zeros(size(mu_p, 1), size(y_hat, 1));

for jj = 1:size(x_p, 2)
    E_y = E_y + w_p(jj)*(y_fake(jj, :)' - y_hat) * (y_fake(jj, :)' - y_hat)';
    E_xy = E_xy + w_p(jj) * (x_p(:, jj) - mu_p) * (y_fake(jj, :)' - y_hat)';
end
E_y = E_y + Rt;

mu_upd = mu_p + E_xy * E_y^(-1) * (yt - y_hat);
sigma_upd = sigma_p - E_xy * E_y^(-1) * E_xy';

mu_upd(1:4) = mu_upd(1:4) ./ norm(mu_upd(1:4));

mu_prev = mu_upd;
sigma_prev = sigma_upd;

end
